simulink subsystem "LQR"  (R2024a)
settings: Solver=VariableStepAuto  StartTime=0.0  StopTime=10.0  RelTol=1e-3
values from neighbouring files (symbols this model uses):
  LQR = [-990.195679828 -22.8679308793 5.6222211134 0.811904406731]    [LQR.mat]
undefined symbols (not defined in the file or in its folder): u_eq, x_eq
settings Model: Creator=Bocchio  LastModifiedBy=Bocchio

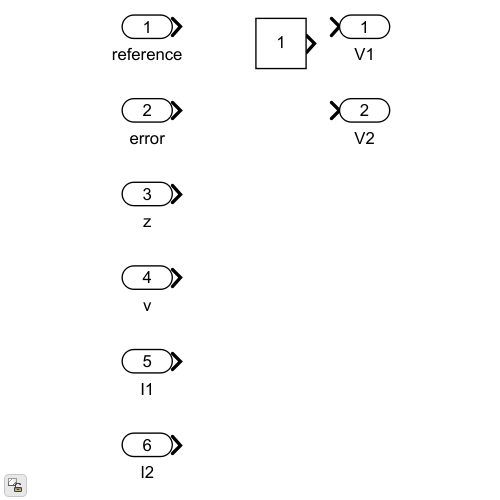
[thumbnail: Simulink's stored preview of the top-level diagram]
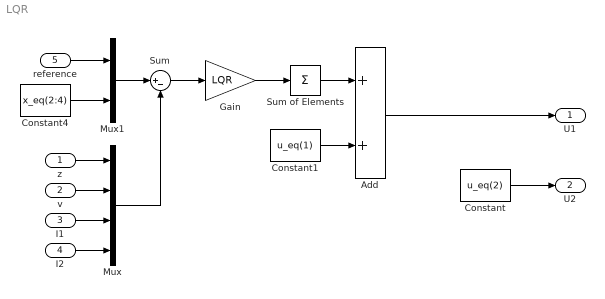
== system LQR ==
  z : Inport
  v : Inport  Port=2
  I1 : Inport  Port=3
  I2 : Inport  Port=4
  reference : Inport  Port=5
  Add : Sum
  Constant : Constant  Value=u_eq(2)
  Constant1 : Constant  Value=u_eq(1)
  Constant4 : Constant  Value=x_eq(2:4)
  Gain : Gain  Gain=LQR
  Mux : Mux
  Mux1 : Mux  Inputs=2
  Sum : Sum  Inputs=|+-
  Sum of Elements : Sum  Inputs=+
  U1 : Outport
  U2 : Outport  Port=2
  wires:
  Constant/1 -> U2/1
  Gain/1 -> Sum of Elements/1
  Add/1 -> U1/1
  Constant1/1 -> Add/2
  Constant4/1 -> Mux1/2
  z/1 -> Mux/1
  v/1 -> Mux/2
  I1/1 -> Mux/3
  I2/1 -> Mux/4
  reference/1 -> Mux1/1
  Sum/1 -> Gain/1
  Mux1/1 -> Sum/1
  Mux/1 -> Sum/2
  Sum of Elements/1 -> Add/1
